simulink model "hw12_feedbackControl"  (R2020a)
settings: Solver=VariableStepAuto  StartTime=0.0  StopTime=30  RelTol=1e-8
undefined symbols (not defined in the file or in its folder): A, B, C, D, IC_ss, K
settings Model: Creator=Tomo  LastModifiedBy=Tomo

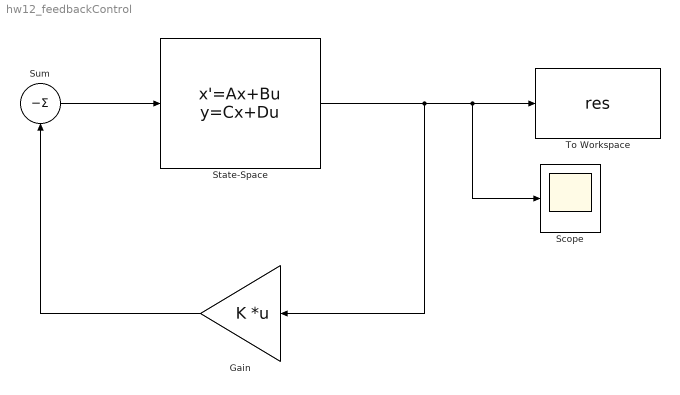
== system hw12_feedbackControl ==
  Gain : Gain  Gain=K  Multiplication=Matrix(K*u)
  Scope : Scope
  State-Space : StateSpace  A=A  B=B  C=C  D=D  InitialCondition=IC_ss
  Sum : Sum  Inputs=|-
  To Workspace : ToWorkspace  VariableName=res  SaveFormat=Structure With Time  SampleTime=-1
  wires:
  State-Space/1 -> Gain/1, Scope/1, To Workspace/1
  Sum/1 -> State-Space/1
  Gain/1 -> Sum/1
